simulink model "UnderactuatedBike"  (R2018b)
settings: Solver=VariableStepAuto  StartTime=0.0  StopTime=50  MaxStep=0.01  RelTol=1e-3
undefined symbols (not defined in the file): A, B, C
libraries: simulink x1
settings Model: Creator=Philip  LastModifiedBy=User
settings DebuggingCC: LibraryContextMissingDiagnostic=none
settings SFSimCC: SimUseLocalCustomCode=off
settings RTWCC: RTWUseLocalCustomCode=off

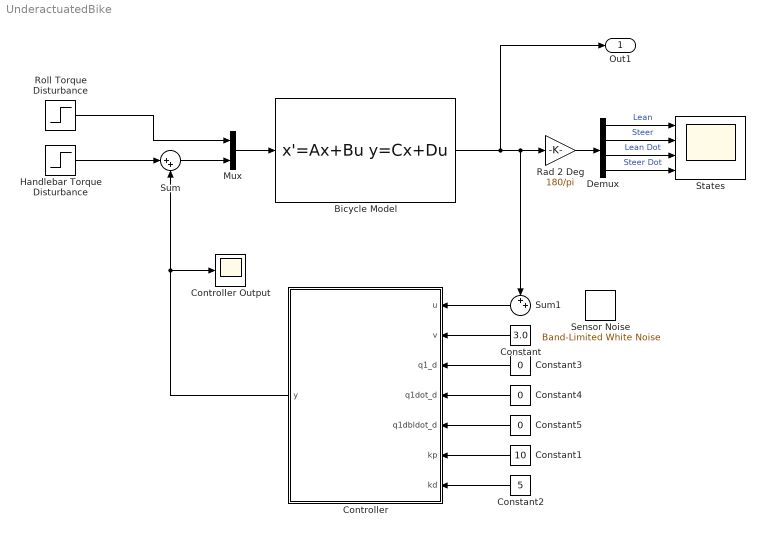
== system UnderactuatedBike ==
  Bicycle Model : StateSpace  A=A  B=B  C=C  D=zeros(4,2)  InitialCondition=0
  Constant : Constant  Value=3.0
  Constant1 : Constant  Value=10
  Constant2 : Constant  Value=5
  Constant3 : Constant  Value=0
  Constant4 : Constant  Value=0
  Constant5 : Constant  Value=0
  Controller : MATLAB Function  TreatAsAtomicUnit=on
  Controller Output : Scope
  Demux : Demux
  Handlebar Torque Disturbance : Step  Time=10  After=0  SampleTime=0
  Mux : Mux  Inputs=2
  Rad 2 Deg : Gain  Gain=180/pi
  Roll Torque Disturbance : Step  Time=2  After=0  SampleTime=0
  Sensor Noise : simulink/Sources/Band-Limited White Noise  Cov=1e-9  Ts=0.01  seed=[23341]
  States : Scope  NumInputPorts=4
  Sum : Sum  Inputs=|++
  Sum1 : Sum  Inputs=++|
  Out1 : Outport
  wires:
  Bicycle Model/1 -> Out1/1, Rad 2 Deg/1, Sum1/1
  Constant/1 -> Controller/2(v)
  Constant1/1 -> Controller/6(kp)
  Constant2/1 -> Controller/7(kd)
  Constant3/1 -> Controller/3(q1_d)
  Constant4/1 -> Controller/4(q1dot_d)
  Constant5/1 -> Controller/5(q1dbldot_d)
  Controller/1(y) -> Controller Output/1, Sum/2
  Handlebar Torque Disturbance/1 -> Sum/1
  Demux/1 -> States/1  "Lean"
  Demux/2 -> States/2  "Steer"
  Demux/3 -> States/3  "Lean Dot"
  Demux/4 -> States/4  "Steer Dot"
  Mux/1 -> Bicycle Model/1
  Sum/1 -> Mux/2
  Roll Torque Disturbance/1 -> Mux/1
  Sum1/1 -> Controller/1(u)
  Rad 2 Deg/1 -> Demux/1

== matlab function UnderactuatedBike/Controller ==
  data: u input; y output; v input; q1_d input; q1dot_d input; q1dbldot_d input; kp input; kd input
function y = fcn(u, v, q1_d, q1dot_d, q1dbldot_d, kp, kd)

    M  = [17.6321, 0.7564; 0.7564, 0.2624];
    C1 = v * [0, 8.9630; -0.8482, 1.0916];
    K0 = [-105.4575, -8.6588; -8.6588, -2.7381];
    K2 = [0, 11.1145; 0, 1.0562];
    K = K0 + v * v * K2;

    q1 = u(1); q2 = u(2); q1dot = u(3); q2dot = u(4);

    h1 = C1(1,2) * q2dot;
    h2 = C1(2,1) * q1dot + C1(2,2) * q2dot;
    phi1 = K(1,1) * q1 + K(1,2) * q2;
    phi2 = K(2,1) * q1 + K(2,2) * q2;

    m1bar = M(2,1) - M(2,2) * M(1,1) / M(1,2);
    h1bar = h2 - M(2,2) * h1 / M(1,2);
    phi1bar = phi2 - M(2,2) * phi1 / M(1,2);

    % Underactuated system desired trajectory
    v1 = q1dbldot_d + kd * (q1dot_d - q1dot) + kp * (q1_d - q1);

    % Virtual model control spring and dashpot
    %kspring = 100;
    %lambda = 20; 
    %v1 = 0.5 * sin(q1 / 2) * (4 * kspring * sin(q1 / 2) + lambda * q1dot * cos(q1 / 2));
        
    y = m1bar * v1 + h1bar + phi1bar;
